simulink model "basic_model_22_vscm"  (R2020b)
settings: Solver=FixedStepAuto  StartTime=0.0  StopTime=tStop  FixedStep=tStep  RelTol=1e-3
undefined symbols (not defined in the file): V_amp, V_freq
libraries: powerlib x20, powerlib_meascontrol x4
settings Model: Creator=kacper  LastModifiedBy=kacper

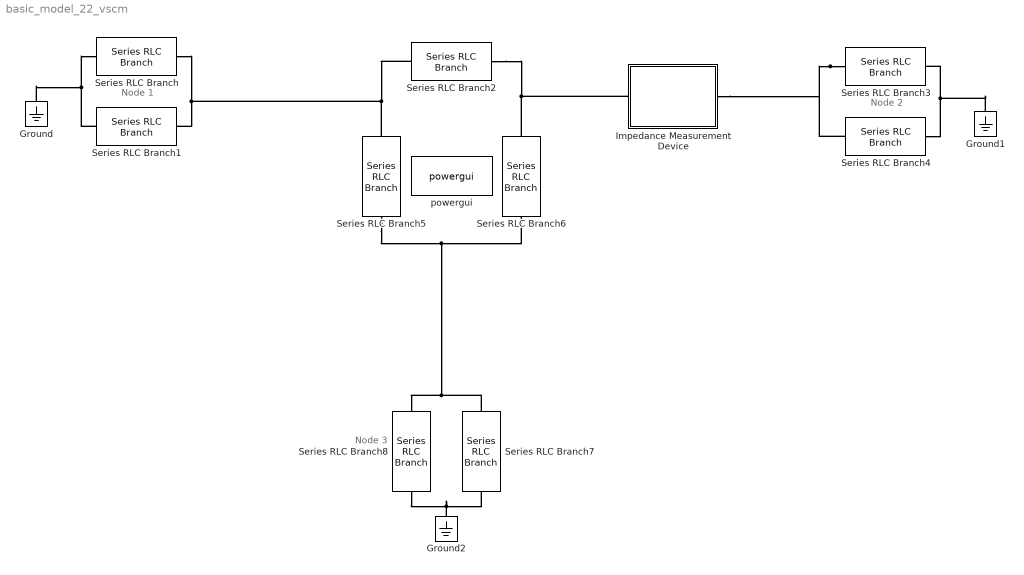
== system basic_model_22_vscm ==
  note: Node 2
  note: Node 1
  note: Node 3
  Ground : powerlib/Elements/Ground  LConnTagsString=a
  Ground1 : powerlib/Elements/Ground  LConnTagsString=a
  Ground2 : powerlib/Elements/Ground  LConnTagsString=a
  Impedance Measurement Device : Subsystem
  Series RLC Branch : powerlib/Elements/Series RLC Branch  LConnTagsString=__new0  RConnTagsString=__new0  BranchType=RL  Resistance=1.2  Inductance=5.8  SetiL0=off  InitialCurrent=0  Capacitance=1e-6  Setx0=off  InitialVoltage=0  Measurements=None
  Series RLC Branch1 : powerlib/Elements/Series RLC Branch  LConnTagsString=__new0  RConnTagsString=__new0  BranchType=C  Resistance=1  Inductance=1e-3  SetiL0=off  InitialCurrent=0  Capacitance=7.9  Setx0=off  InitialVoltage=0  Measurements=None
  Series RLC Branch2 : powerlib/Elements/Series RLC Branch  LConnTagsString=__new0  RConnTagsString=__new0  BranchType=RL  Resistance=0.5  Inductance=0.3  SetiL0=off  InitialCurrent=0  Capacitance=1e-6  Setx0=off  InitialVoltage=0  Measurements=None
  Series RLC Branch3 : powerlib/Elements/Series RLC Branch  LConnTagsString=__new0  RConnTagsString=__new0  BranchType=RL  Resistance=2.2  Inductance=2  SetiL0=off  InitialCurrent=0  Capacitance=1e-6  Setx0=off  InitialVoltage=0  Measurements=None
  Series RLC Branch4 : powerlib/Elements/Series RLC Branch  LConnTagsString=__new0  RConnTagsString=__new0  BranchType=C  Resistance=1  Inductance=1e-3  SetiL0=off  InitialCurrent=0  Capacitance=4  Setx0=off  InitialVoltage=0  Measurements=None
  Series RLC Branch5 : powerlib/Elements/Series RLC Branch  LConnTagsString=__new0  RConnTagsString=__new0  BranchType=RL  Resistance=0.6  Inductance=0.2  SetiL0=off  InitialCurrent=0  Capacitance=1e-6  Setx0=off  InitialVoltage=0  Measurements=None
  Series RLC Branch6 : powerlib/Elements/Series RLC Branch  LConnTagsString=__new0  RConnTagsString=__new0  BranchType=RL  Resistance=1.5  Inductance=0.8  SetiL0=off  InitialCurrent=0  Capacitance=1e-6  Setx0=off  InitialVoltage=0  Measurements=None
  Series RLC Branch7 : powerlib/Elements/Series RLC Branch  LConnTagsString=__new0  RConnTagsString=__new0  BranchType=RL  Resistance=5  Inductance=5  SetiL0=off  InitialCurrent=0  Capacitance=1e-6  Setx0=off  InitialVoltage=0  Measurements=None
  Series RLC Branch8 : powerlib/Elements/Series RLC Branch  LConnTagsString=__new0  RConnTagsString=__new0  BranchType=C  Resistance=1  Inductance=1e-3  SetiL0=off  InitialCurrent=0  Capacitance=6  Setx0=off  InitialVoltage=0  Measurements=None
  powergui : powerlib/powergui  Priority=1  SimulationMode=Continuous  SampleTime=50e-6  frequency=60  Iterations=50  frequencyindice=10000  Pbase=100e6  ErrMax=1e-4  UnitsV=kV  UnitsW=MW  buscounter=0  FunctionMessages=off  echomessages=off  EnableUseOfTLC=off  CurrentSourceSwitches=off  DisableSnubberDevices=off  DisableRonSwitches=off  DisableVfSwitches=off  DisplayEquations=off  AutomaticDiscreteSolvers=off  SolverType=Tustin/Backward Euler (TBE)  Interpol=off  ExternalGateDelay=off  methode=off  Ts=100  x0status=blocks  SPID=on  SwTol=0  HookPort=off  NonlinearTolerance=1e-4  nMaxIteration=100  ContinueOnMaxIteration=off  RestoreLinks=warning  ResistiveCurrentMeasurement=off  Frange=[0:2:500]  Ylog=off  Xlog=on  ShowGrid=off  save=off  variable=ZData  structure=0  ZoomFFT=off  StartTime=0.0  cycles=1  DisplayStyle=1  fundamental=60  FreqAxis=off  MaxFrequency=1000  frequencyindicesteady=1  RmsSteady=1  display=off
  connections:
  Series RLC Branch1/RConn1 -- Series RLC Branch/RConn1 -- Ground/LConn1
  Series RLC Branch2/LConn1 -- Impedance Measurement Device/LConn1 -- Series RLC Branch6/LConn1
  Series RLC Branch4/RConn1 -- Series RLC Branch3/RConn1 -- Ground1/LConn1
  Series RLC Branch2/RConn1 -- Series RLC Branch/LConn1 -- Series RLC Branch1/LConn1 -- Series RLC Branch5/LConn1
  Series RLC Branch8/RConn1 -- Ground2/LConn1 -- Series RLC Branch7/RConn1
  Series RLC Branch5/RConn1 -- Series RLC Branch7/LConn1 -- Series RLC Branch8/LConn1 -- Series RLC Branch6/RConn1
  Series RLC Branch3/LConn1 -- Impedance Measurement Device/RConn1 -- Series RLC Branch4/LConn1

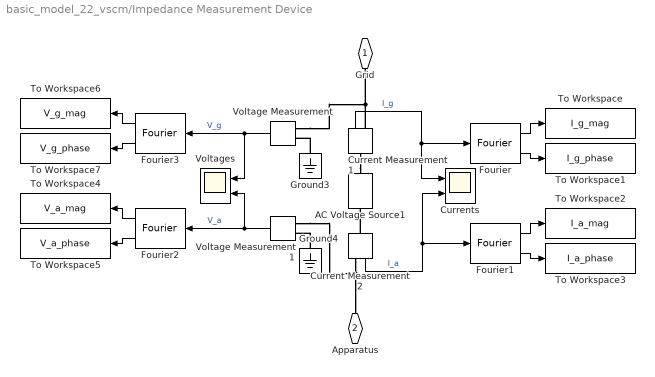
== system basic_model_22_vscm/Impedance Measurement Device ==
  AC Voltage Source1 : powerlib/Electrical Sources/AC Voltage Source  Amplitude=V_amp  Phase=0  Frequency=V_freq  SampleTime=0  Measurements=None  BusType=swing  Pref=10e3  Qref=0  Qmin=-inf  Qmax=+inf
  Current Measurement1 : powerlib/Measurements/Current Measurement  PhasorSimulation=off  OutputType=Complex  PSBequivalent=0
  Current Measurement2 : powerlib/Measurements/Current Measurement  PhasorSimulation=off  OutputType=Complex  PSBequivalent=0
  Currents : Scope  NumInputPorts=2
  Fourier{,1..3} (4 alike) : powerlib_meascontrol/Measurements/Fourier  Freq=V_freq  n=1  InInit=[0, 0]  Ts=0
  Ground3 : powerlib/Elements/Ground  LConnTagsString=a
  Ground4 : powerlib/Elements/Ground  LConnTagsString=a
  To Workspace : ToWorkspace  VariableName=I_g_mag  SampleTime=-1
  To Workspace1 : ToWorkspace  VariableName=I_g_phase  SampleTime=-1
  To Workspace2 : ToWorkspace  VariableName=I_a_mag  SampleTime=-1
  To Workspace3 : ToWorkspace  VariableName=I_a_phase  SampleTime=-1
  To Workspace4 : ToWorkspace  VariableName=V_a_mag  SampleTime=-1
  To Workspace5 : ToWorkspace  VariableName=V_a_phase  SampleTime=-1
  To Workspace6 : ToWorkspace  VariableName=V_g_mag  SampleTime=-1
  To Workspace7 : ToWorkspace  VariableName=V_g_phase  SampleTime=-1
  Voltage Measurement : powerlib/Measurements/Voltage Measurement  PhasorSimulation=off  OutputType=Complex  PSBequivalent=0
  Voltage Measurement1 : powerlib/Measurements/Voltage Measurement  PhasorSimulation=off  OutputType=Complex  PSBequivalent=0
  Voltages : Scope  NumInputPorts=2
  Grid : PMIOPort  Side=Left
  Apparatus : PMIOPort  Port=2  Side=Right
  wires:
  Voltage Measurement1/1 -> Fourier2/1, Voltages/2  "V_a"
  Fourier1/1 -> To Workspace2/1
  Fourier3/2 -> To Workspace7/1
  Fourier/1 -> To Workspace/1
  Fourier/2 -> To Workspace1/1
  Current Measurement2/1 -> Fourier1/1, Currents/2  "I_a"
  Current Measurement1/1 -> Fourier/1, Currents/1  "I_g"
  Fourier3/1 -> To Workspace6/1
  Voltage Measurement/1 -> Fourier3/1, Voltages/1  "V_g"
  Fourier1/2 -> To Workspace3/1
  Fourier2/1 -> To Workspace4/1
  Fourier2/2 -> To Workspace5/1
  connections:
  Voltage Measurement1/LConn1 -- Current Measurement2/RConn1 -- Apparatus/RConn1
  Ground4/LConn1 -- Voltage Measurement1/LConn2
  Current Measurement2/LConn1 -- AC Voltage Source1/LConn1
  Ground3/LConn1 -- Voltage Measurement/LConn2
  Current Measurement1/RConn1 -- Voltage Measurement/LConn1 -- Grid/RConn1
  Current Measurement1/LConn1 -- AC Voltage Source1/RConn1
